simulink model "SimpleMass"  (R2018a)
settings: Solver=FixedStepAuto  StartTime=0.0  StopTime=Ttot  FixedStep=Ts  MaxStep=0.1  RelTol=1e-3
values from neighbouring files (symbols this model uses):
  bat = []    [SimpleMass_Script.m]
  fc = []    [SimpleMass_Script.m]
  Fn = 50    [SimpleMass_Script.m]
  gov = []    [SimpleMass_Script.m]
  J = 2 * H * Sn / omegan^2    (= 4458.13208026)    [SimpleMass_Script.m]
  load = []    [SimpleMass_Script.m]
  omegan = 2 * pi * Fn / np    (= 314.159265359)    [SimpleMass_Script.m]
  Sn = 2*44e6    (= 88000000)    [SimpleMass_Script.m]
  wf = []    [SimpleMass_Script.m]
undefined symbols (not defined in the file or in its folder): sec
settings Model: Creator=daniemot  LastModifiedBy=daniemot

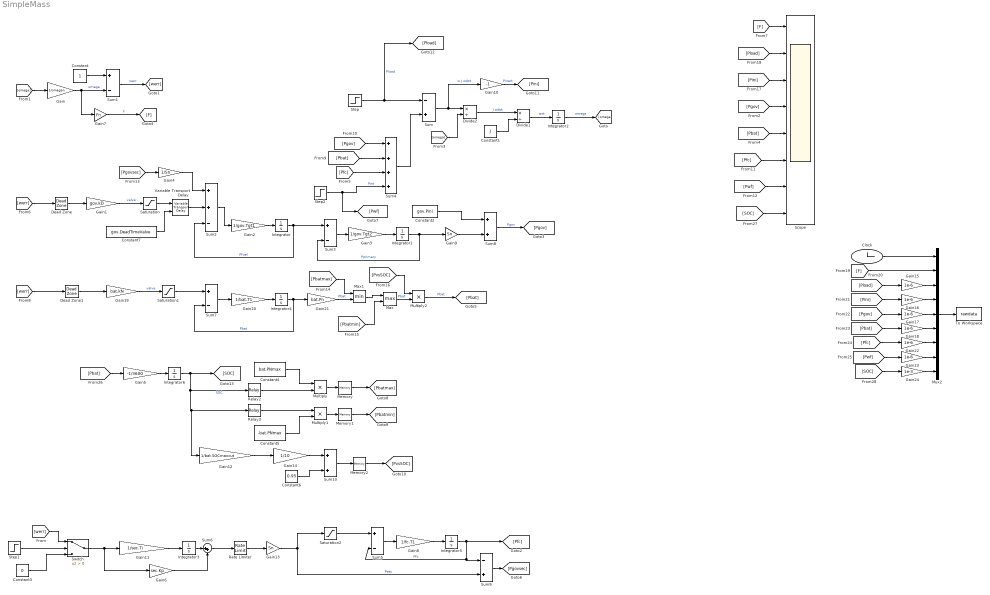
== system SimpleMass ==
  Clock : Clock
  Constant : Constant
  Constant1 : Constant  Value=J
  Constant2 : Constant  Value=gov.Pini
  Constant3 : Constant  Value=0
  Constant4 : Constant  Value=bat.PNmax
  Constant5 : Constant  Value=-bat.PNmax
  Constant6 : Constant  Value=0.95
  Constant7 : Constant  Value=gov.DeadTimeValve
  Dead Zone : DeadZone  LowerValue=-gov.fD  UpperValue=gov.fD  SaturateOnIntegerOverflow=on
  Dead Zone1 : DeadZone  LowerValue=-bat.fN  UpperValue=bat.fN  SaturateOnIntegerOverflow=on
  Divide1 : Product  Inputs=*/
  Divide2 : Product  Inputs=*/
  Gain : Gain  Gain=1/omegan
  Gain1 : Gain  Gain=gov.kD
  Gain10 : Gain  Gain=-1
  Gain11 : Gain  Gain=1/sec.Ti
  Gain12 : Gain  Gain=1/bat.SOCmaxcut
  Gain13 : Gain  Gain=Sn
  Gain14 : Gain  Gain=1/10
  Gain{15..18,22..23} (6 alike) : Gain  Gain=1e-6
  Gain19 : Gain  Gain=bat.kN
  Gain2 : Gain  Gain=1/gov.Tgt1
  Gain20 : Gain  Gain=1/bat.T1
  Gain21 : Gain  Gain=bat.Pn
  Gain24 : Gain  Gain=1e-3
  Gain3 : Gain  Gain=1/gov.Tgt2
  Gain4 : Gain  Gain=1/Sn
  Gain5 : Gain  Gain=-1/3600
  Gain6 : Gain  Gain=sec.Kp
  Gain7 : Gain  Gain=Fn
  Gain8 : Gain  Gain=1/fc.T1
  Gain9 : Gain  Gain=Sn
  Integrator{,1,3..5} (5 alike) : Integrator
  Integrator2 : Integrator  InitialCondition=omegan
  Integrator6 : Integrator  InitialCondition=bat.SOCini
  Max : MinMax  Function=max  Inputs=2
  Max1 : MinMax  Inputs=2
  Memory : Memory  InitialCondition=bat.PNmax
  Memory1 : Memory  InitialCondition=-bat.PNmax
  Memory2 : Memory  InitialCondition=0.1*bat.SOCini/bat.SOCmaxcut+0.95
  Multiply : Product
  Multiply1 : Product
  Multiply2 : Product
  Mux2 : Mux  Inputs=9
  Rate Limiter : RateLimiter  RisingSlewLimit=sec.Rate  FallingSlewLimit=-sec.Rate  SampleTimeMode=inherited
  Relay2 : Relay  OnSwitchValue=bat.SOCminrest  OffSwitchValue=bat.SOCmincut
  Relay3 : Relay  OnSwitchValue=bat.SOCmaxcut  OffSwitchValue=bat.SOCmaxrest  OnOutputValue=0  OffOutputValue=1
  Saturation : Saturate  UpperLimit=gov.pDmax  LowerLimit=-gov.pDmax
  Saturation1 : Saturate  UpperLimit=bat.pNmax  LowerLimit=-bat.pNmax
  Saturation2 : Saturate  UpperLimit=fc.Pmax  LowerLimit=0
  Scope : Scope  NumInputPorts=8
  Step : Step  Time=load.StepTime  Before=load.Pini  After=load.Pini + load.Pstep  SampleTime=0
  Step1 : Step  Time=sec.T_on_delay  SampleTime=0
  Step2 : Step  Time=wf.StepTime  Before=wf.Pini  After=wf.Pini + wf.Pstep  SampleTime=0
  Sum : Sum  Inputs=-+
  Sum{1,3,5,7} (4 alike) : Sum  Inputs=+-
  Sum10 : Sum
  Sum2 : Sum  Inputs=++-
  Sum4 : Sum  Inputs=++++
  Sum6 : Sum  Inputs=|++
  Sum8 : Sum
  Sum9 : Sum  Inputs=-+
  Switch : Switch  Criteria=u2 > Threshold
  To Workspace : ToWorkspace  VariableName=rawdata  SampleTime=-1
  Variable Transport Delay : VariableTransportDelay  VariableDelayType=Variable transport delay  MaximumDelay=10  MaximumPoints=4096
  wires:
  [omega] -> Gain/1
  Gain/1 -> Gain7/1, Sum1/2  "omega"
  Constant/1 -> Sum1/1
  Sum1/1 -> [werr]  "werr"
  Gain1/1 -> Saturation/1  "valve"
  Gain2/1 -> Integrator/1
  Sum2/1 -> Gain2/1
  Integrator1/1 -> Gain9/1, Sum3/2  "Pprimary"
  Integrator/1 -> Sum2/3, Sum3/1  "Pfuel"
  Gain3/1 -> Integrator1/1
  Sum3/1 -> Gain3/1
  Step/1 -> [Pload], Sum/1  "Pload"
  Divide2/1 -> Divide1/1  "J wdot"
  Constant1/1 -> Divide1/2
  Divide1/1 -> Integrator2/1  "wot"
  Integrator2/1 -> [omega]  "omega"
  [omega] -> Divide2/2
  Sum/1 -> Gain10/1, Divide2/1  "w J wdot"
  Variable Transport Delay/1 -> Sum2/2
  Constant7/1 -> Variable Transport Delay/2
  Sum8/1 -> [Pgov]  "Pgov"
  Gain11/1 -> Integrator3/1
  Sum6/1 -> Rate Limiter/1
  Gain10/1 -> [Pini]  "Pinert"
  Gain13/1 -> Sum9/2, Saturation2/1  "Psec"
  Integrator3/1 -> Sum6/1
  Step1/1 -> Switch/2
  Constant3/1 -> Switch/3
  Mux2/1 -> To Workspace/1
  Clock/1 -> Mux2/1
  Switch/1 -> Gain11/1, Gain6/1
  Gain6/1 -> Sum6/2
  [werr] -> Switch/1
  [werr] -> Dead Zone/1
  Dead Zone/1 -> Gain1/1
  Saturation/1 -> Variable Transport Delay/1
  [werr] -> Dead Zone1/1
  Dead Zone1/1 -> Gain19/1
  Integrator4/1 -> Gain21/1, Sum7/2  "Pbat"
  Gain20/1 -> Integrator4/1
  Gain19/1 -> Saturation1/1  "valve"
  Sum7/1 -> Gain20/1
  Saturation1/1 -> Sum7/1
  Multiply2/1 -> [Pbat]  "Pbat"
  [Pgov] -> Sum4/1
  [Pbat] -> Sum4/2
  [Pfc] -> Sum4/3
  Sum4/1 -> Sum/2
  [Pgov] -> Scope/4
  [Pfc] -> Scope/6
  Saturation2/1 -> Sum5/1
  Integrator5/1 -> Sum5/2, Sum9/1, [Pfc]  "Pfc"
  [Pgovsec] -> Gain4/1
  Gain4/1 -> Sum2/1
  Gain8/1 -> Integrator5/1
  Sum5/1 -> Gain8/1
  Sum9/1 -> [Pgovsec]
  Step2/1 -> [Pwf], Sum4/4  "Pwt"
  [Pwf] -> Scope/7
  Gain9/1 -> Sum8/2
  Constant2/1 -> Sum8/1
  Gain5/1 -> Integrator6/1
  Rate Limiter/1 -> Gain13/1
  Constant4/1 -> Multiply/1
  Constant5/1 -> Multiply1/2
  Multiply/1 -> Memory/1
  Multiply1/1 -> Memory1/1
  Memory1/1 -> [Pbatmin]
  Memory/1 -> [Pbatmax]
  Gain21/1 -> Max1/2  "Pbat"
  [Pbatmax] -> Max1/1
  [Pbatmin] -> Max/2
  Max1/1 -> Max/1
  Integrator6/1 -> [SOC], Gain12/1, Relay3/1, Relay2/1  "SOC"
  Relay2/1 -> Multiply/2
  Relay3/1 -> Multiply1/1
  Gain12/1 -> Gain14/1
  Gain14/1 -> Sum10/1
  Constant6/1 -> Sum10/2
  Sum10/1 -> Memory2/1
  Max/1 -> Multiply2/2  "Pbat"
  [PvsSOC] -> Multiply2/1
  Memory2/1 -> [PvsSOC]
  [Pini] -> Scope/3
  Gain7/1 -> [F]  "F"
  [F] -> Scope/1
  [Pload] -> Scope/2
  [Pbat] -> Scope/5
  [F] -> Mux2/2
  [Pload] -> Gain15/1
  [Pini] -> Gain16/1
  [Pgov] -> Gain17/1
  [Pbat] -> Gain18/1
  [Pfc] -> Gain22/1
  [Pwf] -> Gain23/1
  [Pbat] -> Gain5/1
  [SOC] -> Scope/8
  [SOC] -> Gain24/1
  Gain15/1 -> Mux2/3
  Gain16/1 -> Mux2/4
  Gain17/1 -> Mux2/5
  Gain18/1 -> Mux2/6
  Gain22/1 -> Mux2/7
  Gain23/1 -> Mux2/8
  Gain24/1 -> Mux2/9
